simulink model "modeledelexperience"  (R2018b)
settings: Solver=VariableStepAuto  StartTime=0.0  StopTime=50  RelTol=1e-3  EnableMultiTasking=on
libraries: fl_lib x21, nesl_utility x10
settings Model: Creator=arnalg  LastModifiedBy=TRABETC
settings DataIOCC: LimitDataPoints=on  SaveFormat=Array  SignalLoggingSaveFormat=ModelDataLogs
settings OptimizationCC: ExpressionDepthLimit=2147483647  LifeSpan=inf
settings DebuggingCC: UnderspecifiedInitializationDetection=Classic  MergeDetectMultiDrivingBlocksExec=none  SolverPrmCheckMsg=warning  FcnCallInpInsideContextMsg=warning  StateNameClashWarn=warning  SFUnexpectedBacktrackingDiag=warning  SFNoUnconditionalDefaultTransitionDiag=warning  SFExecutionAtInitializationDiag=none
settings HardwareCC: ProdBitPerPointer=32  ProdBitPerSizeT=32  ProdBitPerPtrDiffT=32  ProdLargestAtomicFloat=None  ProdIntDivRoundTo=Undefined  ProdEndianess=Unspecified  ProdWordSize=32  ProdHWDeviceType=32-bit Generic
settings ModelReferenceCC: PropagateSignalLabelsOutOfModel=off
settings SFSimCC: SimUseLocalCustomCode=off
settings RTWCC: RTWUseLocalCustomCode=off
settings CodeAppCC: StateflowObjectComments=on
settings GRTTargetCC: TargetLangStandard=C89/C90 (ANSI)  GeneratePreprocessorConditionals=Disable all  CombineOutputUpdateFcns=off  GRTInterface=on
settings ConfigComp: CovMetricSettings=dw  CovHtmlReporting=on  CovSaveCumulativeToWorkspaceVar=on  CovSaveSingleToWorkspaceVar=on  CovExternalEMLEnable=off
settings SimscapeCC: SimscapeNormalizeSystem=off

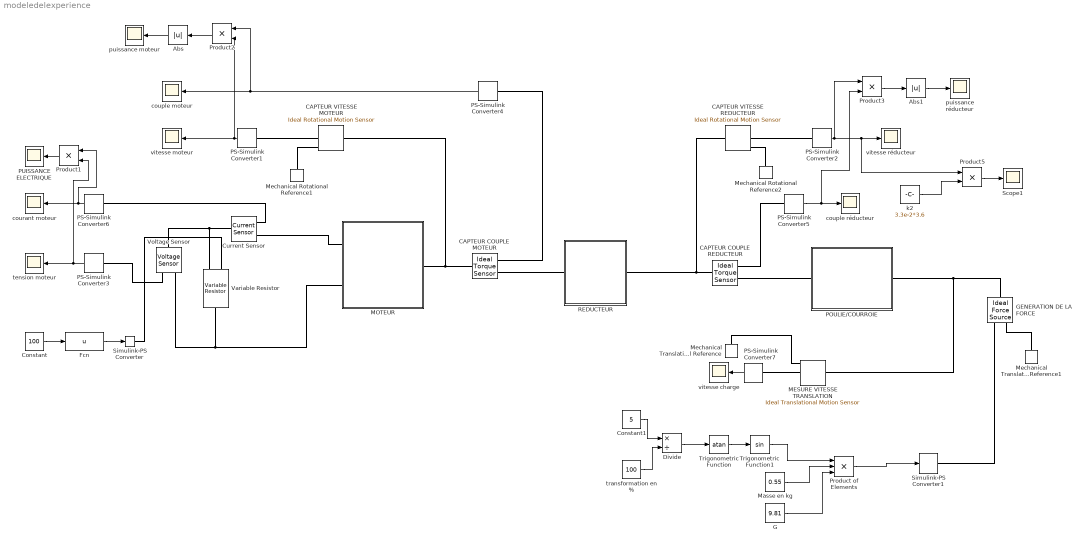
== system modeledelexperience ==
  Abs : Abs
  Abs1 : Abs
  CAPTEUR COUPLE MOTEUR : fl_lib/Mechanical/Mechanical Sensors/Ideal Torque Sensor
  CAPTEUR VITESSE MOTEUR : fl_lib/Mechanical/Mechanical Sensors/Ideal Rotational Motion Sensor  offset=0 rad
  CAPTEUR VITESSE REDUCTEUR : fl_lib/Mechanical/Mechanical Sensors/Ideal Rotational Motion Sensor  offset=0 rad
  CAPTEUR COUPLE REDUCTEUR : fl_lib/Mechanical/Mechanical Sensors/Ideal Torque Sensor
  Constant : Constant  Value=100
  Constant1 : Constant  Value=5
  Current Sensor : fl_lib/Electrical/Electrical Sensors/Current Sensor
  Divide : Product  Inputs=*/
  Fcn : Fcn  Expr=u
  G : Constant  Value=9.81
  GENERATION DE LA FORCE : fl_lib/Mechanical/Mechanical Sources/Ideal Force Source
  MESURE VITESSE TRANSLATION : fl_lib/Mechanical/Mechanical Sensors/Ideal Translational Motion Sensor  offset=0 m
  MOTEUR : Subsystem
  Masse en kg : Constant  Value=0.55
  Mechanical Rotational Reference1 : fl_lib/Mechanical/Rotational Elements/Mechanical Rotational Reference
  Mechanical Rotational Reference2 : fl_lib/Mechanical/Rotational Elements/Mechanical Rotational Reference
  Mechanical Translational Reference : fl_lib/Mechanical/Translational Elements/Mechanical Translational Reference
  Mechanical Translational Reference1 : fl_lib/Mechanical/Translational Elements/Mechanical Translational Reference
  POULIE/COURROIE : Subsystem
  PS-Simulink Converter{1..7} (7 alike) : nesl_utility/PS-Simulink Converter  PhysicalDomain=network_engine_domain  SubClassName=ps_output  LeftPortType=input  RightPortType=output  PseudoPeriodic=off  Frequencies=[]  Unit=1  AffineConversion=off
  PUISSANCE ELECTRIQUE : Scope
  Product of Elements : Product  Inputs=3
  Product{1..3,5} (4 alike) : Product
  REDUCTEUR : Subsystem
  Scope1 : Scope
  Simulink-PS Converter : nesl_utility/Simulink-PS Converter  PhysicalDomain=network_engine_domain  SubClassName=ps_input  LeftPortType=input  RightPortType=output  PseudoPeriodic=off  Frequencies=[]  NoiseDistribution=none  NoiseParameters=[]  Unit=1  AffineConversion=off  FilteringAndDerivatives=provide  SimscapeFilterOrder=1  InputFilterTimeConstant=0.001  UdotUserProvided=0
  Simulink-PS Converter1 : nesl_utility/Simulink-PS Converter  PhysicalDomain=network_engine_domain  SubClassName=ps_input  LeftPortType=input  RightPortType=output  PseudoPeriodic=off  Frequencies=[]  NoiseDistribution=none  NoiseParameters=[]  Unit=1  AffineConversion=off  FilteringAndDerivatives=zero  SimscapeFilterOrder=1  InputFilterTimeConstant=.001  UdotUserProvided=0
  Trigonometric Function : Trigonometry  Operator=atan
  Trigonometric Function1 : Trigonometry
  Variable Resistor : fl_lib/Electrical/Electrical Elements/Variable Resistor  Rmin=0 Ohm  i_specify=off  i_priority=None  i=0 A  i_nominal_specify=off  i_nominal_unit=A  i_nominal_value=1  v_specify=off  v_priority=None  v=0 V  v_nominal_specify=off  v_nominal_unit=V  v_nominal_value=1
  Voltage Sensor : fl_lib/Electrical/Electrical Sensors/Voltage Sensor
  couple moteur : Scope
  couple réducteur : Scope
  courant moteur : Scope
  k2 : Constant  Value=3.3e-2*3.6
  puissance moteur : Scope
  puissance réducteur : Scope
  tension moteur : Scope
  transformation en % : Constant  Value=100
  vitesse charge : Scope
  vitesse moteur : Scope
  vitesse réducteur : Scope
  wires:
  PS-Simulink Converter1/1 -> Product2/2, vitesse moteur/1
  PS-Simulink Converter7/1 -> vitesse charge/1
  PS-Simulink Converter5/1 -> Product3/2, couple réducteur/1
  PS-Simulink Converter6/1 -> Product1/1, courant moteur/1
  PS-Simulink Converter4/1 -> Product2/1, couple moteur/1
  Product2/1 -> Abs/1
  Product3/1 -> Abs1/1
  Abs/1 -> puissance moteur/1
  Abs1/1 -> puissance réducteur/1
  Product1/1 -> PUISSANCE ELECTRIQUE/1
  Constant1/1 -> Divide/1
  transformation en %/1 -> Divide/2
  Divide/1 -> Trigonometric Function/1
  Masse en kg/1 -> Product of Elements/2
  G/1 -> Product of Elements/3
  Product5/1 -> Scope1/1
  k2/1 -> Product5/2
  Product of Elements/1 -> Simulink-PS Converter1/1
  Trigonometric Function1/1 -> Product of Elements/1
  Trigonometric Function/1 -> Trigonometric Function1/1
  PS-Simulink Converter2/1 -> Product3/1, Product5/1, vitesse réducteur/1
  PS-Simulink Converter3/1 -> tension moteur/1, Product1/2
  Fcn/1 -> Simulink-PS Converter/1
  Constant/1 -> Fcn/1
  connections:
  Mechanical Rotational Reference1/LConn1 -- CAPTEUR VITESSE MOTEUR/RConn1
  Voltage Sensor/RConn1 -- PS-Simulink Converter3/LConn1
  CAPTEUR VITESSE MOTEUR/RConn2 -- PS-Simulink Converter1/LConn1
  Current Sensor/LConn1 -- Voltage Sensor/LConn1 -- Variable Resistor/LConn2
  Current Sensor/RConn1 -- PS-Simulink Converter6/LConn1
  Mechanical Rotational Reference2/LConn1 -- CAPTEUR VITESSE REDUCTEUR/RConn1
  CAPTEUR VITESSE REDUCTEUR/RConn2 -- PS-Simulink Converter2/LConn1
  MESURE VITESSE TRANSLATION/LConn1 -- GENERATION DE LA FORCE/LConn1 -- POULIE/COURROIE/RConn1
  MESURE VITESSE TRANSLATION/RConn2 -- PS-Simulink Converter7/LConn1
  GENERATION DE LA FORCE/RConn1 -- Simulink-PS Converter1/RConn1
  Mechanical Translational Reference1/LConn1 -- GENERATION DE LA FORCE/RConn2
  MESURE VITESSE TRANSLATION/RConn1 -- Mechanical Translational Reference/LConn1
  CAPTEUR COUPLE MOTEUR/LConn1 -- CAPTEUR VITESSE MOTEUR/LConn1 -- MOTEUR/RConn1
  CAPTEUR COUPLE MOTEUR/RConn2 -- PS-Simulink Converter4/LConn1
  PS-Simulink Converter5/LConn1 -- CAPTEUR COUPLE REDUCTEUR/RConn2
  Voltage Sensor/RConn2 -- MOTEUR/LConn2 -- Variable Resistor/RConn1
  Current Sensor/RConn2 -- MOTEUR/LConn1
  CAPTEUR COUPLE REDUCTEUR/LConn1 -- CAPTEUR VITESSE REDUCTEUR/LConn1 -- REDUCTEUR/RConn1
  CAPTEUR COUPLE MOTEUR/RConn1 -- REDUCTEUR/LConn1
  CAPTEUR COUPLE REDUCTEUR/RConn1 -- POULIE/COURROIE/LConn1
  Simulink-PS Converter/RConn1 -- Variable Resistor/LConn1

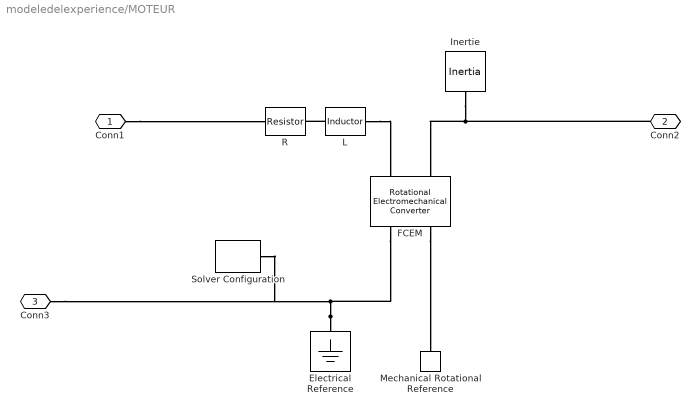
== system modeledelexperience/MOTEUR ==
  Electrical Reference : fl_lib/Electrical/Electrical Elements/Electrical Reference
  FCEM : fl_lib/Electrical/Electrical Elements/Rotational Electromechanical Converter  K=4.15e-3 V/(rad/s)  i_specify=off  i_priority=None  i=0 A  i_nominal_specify=off  i_nominal_unit=A  i_nominal_value=1  v_specify=off  v_priority=None  v=0 V  v_nominal_specify=off  v_nominal_unit=V  v_nominal_value=1  t_specify=off  t_priority=None  t=0 N*m  t_nominal_specify=off  t_nominal_unit=N*m  t_nominal_value=1  w_specify=off  w_priority=None  w=0 rad/s  w_nominal_specify=off  w_nominal_unit=rad/s  w_nominal_value=1
      settings: AttributesFormatString="K = %<K>  %<K_unit>"  SourceProductName=Simscape
  Inertie : fl_lib/Mechanical/Rotational Elements/Inertia  inertia=20 g*cm^2  w_specify=on  w_priority=High  w=0 rad/s  w_nominal_specify=off  w_nominal_unit=rad/s  w_nominal_value=1  t_specify=off  t_priority=None  t=0 N*m  t_nominal_specify=off  t_nominal_unit=N*m  t_nominal_value=1
      settings: AttributesFormatString=J = %<inertia> %<inertia_unit>
  L : fl_lib/Electrical/Electrical Elements/Inductor  l=8 mH  r=0 Ohm  g=1e-9 1/Ohm  i_specify=off  i_priority=None  i=0 A  i_nominal_specify=off  i_nominal_unit=A  i_nominal_value=1  v_specify=off  v_priority=None  v=0 V  v_nominal_specify=off  v_nominal_unit=V  v_nominal_value=1  i_L_specify=on  i_L_priority=High  i_L=0 A  i_L_nominal_specify=off  i_L_nominal_unit=A  i_L_nominal_value=1
      settings: AttributesFormatString=%<l> %<l_unit>
  Mechanical Rotational Reference : fl_lib/Mechanical/Rotational Elements/Mechanical Rotational Reference
  R : fl_lib/Electrical/Electrical Elements/Resistor  R=5.81 Ohm  i_specify=off  i_priority=None  i=0 A  i_nominal_specify=off  i_nominal_unit=A  i_nominal_value=1  v_specify=off  v_priority=None  v=0 V  v_nominal_specify=off  v_nominal_unit=V  v_nominal_value=1
      settings: AttributesFormatString=%<R> %<R_unit>
  Solver Configuration : nesl_utility/Solver Configuration  PhysicalDomain=network_engine_domain  SubClassName=solver  LeftPortType=input  RightPortType=generic  Tones=[]  Harmonics=[]  SimulateNoise=off  Profile=off  UseLocalSampling=off  EnableSwitchedLinearOptims=on  FrequencyDomain=off  UseCCode=off  RelTol=0.001  AbsTol=1e-06  MinStep=1e-09  ToWorkspace=off  RevertToSquareIcSolve=off  NumHomotopyIterations=100  PhasorMode=off  PhasorModeNumHarmonics=1  DoDC=off  ResidualTolerance=1e-9  UseLocalSolver=off  LocalSolverChoice=NE_BACKWARD_EULER_ADVANCER  LocalSolverSampleTime=.01  DoFixedCost=on  MaxNonlinIter=3  MaxModeIter=2  LinearAlgebra=Sparse  EquationFormulation=NE_TIME_EF  DelaysMemoryBudget=1024  AutomaticFiltering=on  FilteringTimeConstant=0.001  PartitionStorageMethod=AS_NEEDED  PartitionMemoryBudget=1024
  Conn1 : PMIOPort  Side=Left
  Conn2 : PMIOPort  Port=2  Side=Right
  Conn3 : PMIOPort  Port=3  Side=Left
  connections:
  Conn1/RConn1 -- R/LConn1
  FCEM/RConn2 -- Mechanical Rotational Reference/LConn1
  L/RConn1 -- FCEM/LConn1
  Inertie/LConn1 -- Conn2/RConn1 -- FCEM/LConn2
  Electrical Reference/LConn1 -- Conn3/RConn1 -- Solver Configuration/RConn1 -- FCEM/RConn1
  L/LConn1 -- R/RConn1

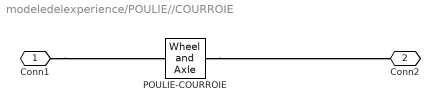
== system modeledelexperience/POULIE//COURROIE ==
  "POULIE-COURROIE " : fl_lib/Mechanical/Mechanisms/Wheel and Axle  R=3.3 cm  or=1  t_specify=off  t_priority=None  t=0 N*m  t_nominal_specify=off  t_nominal_unit=N*m  t_nominal_value=1  f_specify=off  f_priority=None  f=0 N  f_nominal_specify=off  f_nominal_unit=N  f_nominal_value=1
      settings: SourceProductName=Simscape
  Conn1 : PMIOPort  Side=Left
  Conn2 : PMIOPort  Port=2  Side=Right
  connections:
  "POULIE-COURROIE "/RConn1 -- Conn2/RConn1
  Conn1/RConn1 -- "POULIE-COURROIE "/LConn1

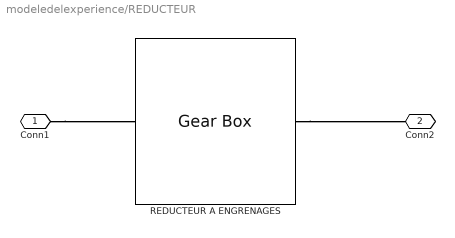
== system modeledelexperience/REDUCTEUR ==
  REDUCTEUR A ENGRENAGES : fl_lib/Mechanical/Mechanisms/Gear Box  ratio=48  t_in_specify=off  t_in_priority=None  t_in=0 N*m  t_in_nominal_specify=off  t_in_nominal_unit=N*m  t_in_nominal_value=1  t_out_specify=off  t_out_priority=None  t_out=0 N*m  t_out_nominal_specify=off  t_out_nominal_unit=N*m  t_out_nominal_value=1
      settings: AttributesFormatString=%<ratio>
  Conn1 : PMIOPort  Side=Left
  Conn2 : PMIOPort  Port=2  Side=Right
  connections:
  Conn1/RConn1 -- REDUCTEUR A ENGRENAGES/LConn1
  REDUCTEUR A ENGRENAGES/RConn1 -- Conn2/RConn1
